simulink model "My747m14ddelay"  (R2021b)
settings: Solver=ode5  StartTime=0.0  StopTime=50  FixedStep=Ts  RelTol=1e-3
values from neighbouring files (symbols this model uses):
  B = B(:,1:2)    [TwoTankSystem.m]
  Ts = 1    [TwoTankSystem.m]
undefined symbols (not defined in the file or in its folder): A, C, Kd, T
settings Model: Creator=tanzc  LastModifiedBy=tanzc
settings DataIOCC: ReturnWorkspaceOutputs=off

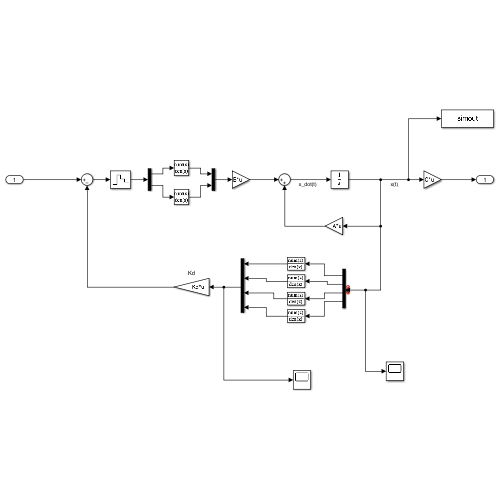
[thumbnail: Simulink's stored preview of the top-level diagram]
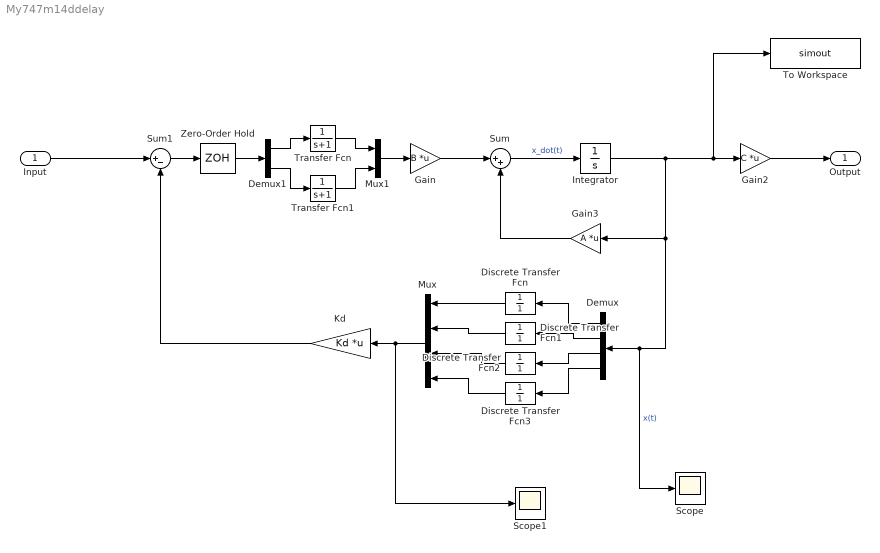
== system My747m14ddelay ==
  Input : Inport  PortDimensions=2
  Demux : Demux
  Demux1 : Demux  Outputs=2
  Discrete Transfer Fcn{,1..3} (4 alike) : DiscreteTransferFcn  Denominator=1  SampleTime=Ts
  Gain : Gain  Gain=B  Multiplication=Matrix(K*u)
  Gain2 : Gain  Gain=C  Multiplication=Matrix(K*u)  OutDataTypeStr=Inherit: Same as input
  Gain3 : Gain  Gain=A  Multiplication=Matrix(K*u)
  Integrator : Integrator
  Kd : Gain  Gain=Kd  Multiplication=Matrix(K*u)  SaturateOnIntegerOverflow=on  SampleTime=T  OutDataTypeStr=Inherit: Same as input  ParamDataTypeStr=Inherit: Same as input
  Mux : Mux
  Mux1 : Mux  Inputs=2
  Scope : Scope
  Scope1 : Scope
  Sum : Sum  Inputs=|++
  Sum1 : Sum  Inputs=|+-  SaturateOnIntegerOverflow=on
  To Workspace : ToWorkspace  VariableName=simout  SampleTime=-1
  Transfer Fcn : TransferFcn  Denominator=[1 1]
  Transfer Fcn1 : TransferFcn  Denominator=[1 1]
  Zero-Order Hold : ZeroOrderHold  SampleTime=Ts
  Output : Outport
  wires:
  Gain/1 -> Sum/1
  Integrator/1 -> Scope/1, Demux/1, Gain3/1, To Workspace/1, Gain2/1  "x(t)"
  Sum/1 -> Integrator/1  "x_dot(t)"
  Gain3/1 -> Sum/2
  Sum1/1 -> Zero-Order Hold/1
  Gain2/1 -> Output/1
  Kd/1 -> Sum1/2
  Input/1 -> Sum1/1
  Discrete Transfer Fcn/1 -> Mux/1
  Discrete Transfer Fcn1/1 -> Mux/2
  Discrete Transfer Fcn2/1 -> Mux/3
  Discrete Transfer Fcn3/1 -> Mux/4
  Demux1/1 -> Transfer Fcn/1
  Zero-Order Hold/1 -> Demux1/1
  Demux1/2 -> Transfer Fcn1/1
  Transfer Fcn1/1 -> Mux1/2
  Transfer Fcn/1 -> Mux1/1
  Mux1/1 -> Gain/1
  Demux/1 -> Discrete Transfer Fcn/1
  Demux/2 -> Discrete Transfer Fcn1/1
  Demux/3 -> Discrete Transfer Fcn2/1
  Demux/4 -> Discrete Transfer Fcn3/1
  Mux/1 -> Scope1/1, Kd/1
